simulink model "sampleModel10"  (R2021a)
settings: Solver=VariableStepAuto  StartTime=0.0  StopTime=10.0  RelTol=1e-3
undefined symbols (not defined in the file): Newton, Raphson
libraries: simulink x16, simulink_need_slupdate x4
settings Model: Creator=user  LastModifiedBy=user

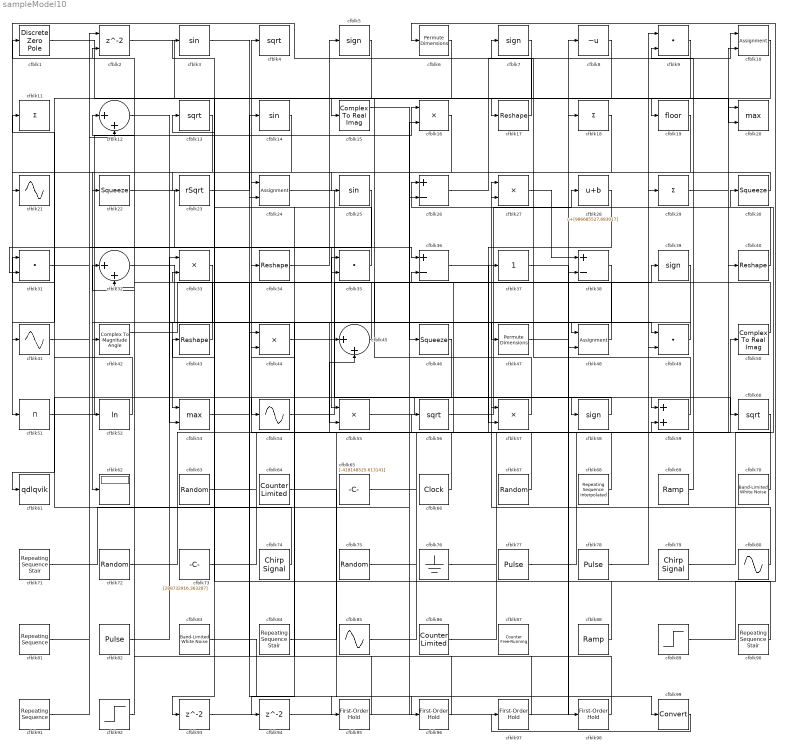
== system sampleModel10 ==
  cfblk1 : DiscreteZeroPole  Poles=[0 0.5]  Gain=1
  cfblk10 : Assignment  DiagnosticForDimensions=Warning  IndexOptions=Index vector (dialog)  Indices=1  OutputSizes=1
  cfblk11 : Sum  Inputs=+
  cfblk12 : Sum  Inputs=|++
  cfblk{4,13,56,60} (4 alike) : Sqrt  SaturateOnIntegerOverflow=on
  cfblk14 : Trigonometry
  cfblk15 : ComplexToRealImag
  cfblk{16,27,33,44,55} (5 alike) : Product
  cfblk{17,34,40,43} (4 alike) : Reshape
  cfblk18 : Sum  Inputs=+
  cfblk19 : Rounding
  cfblk2 : Delay  ShowEnablePort=on  SampleTime=1
      settings: InputPortMap=u0,e6
  cfblk20 : MinMax  Function=max  Inputs=2
  cfblk21 : Sin  TimeSource=Use external signal  SampleTime=0
  cfblk22 : Squeeze
  cfblk23 : Sqrt  Operator=rSqrt  AlgorithmType=Newton-Raphson  SaturateOnIntegerOverflow=on
  cfblk24 : Assignment  DiagnosticForDimensions=Warning  IndexOptions=Index vector (dialog)  Indices=1  OutputSizes=1
  cfblk25 : Trigonometry
  cfblk26 : Sum  Inputs=+-
  cfblk28 : Bias  Bias=[986685527.683017]
  cfblk29 : Sum  Inputs=+
  cfblk3 : Trigonometry
  cfblk30 : Squeeze
  cfblk{9,31,35,49} (4 alike) : DotProduct  InputSameDT=on  OutDataTypeStr=Inherit: Inherit via internal rule
  cfblk32 : Sum  Inputs=|++
  cfblk36 : Sum  Inputs=+-
  cfblk37 : simulink/Math Operations/Slider Gain  gain=1  low=0  high=2
  cfblk38 : Sum  Inputs=+-
  cfblk{5,7,39,58} (4 alike) : Signum
  cfblk41 : Sin  TimeSource=Use external signal  SampleTime=0
  cfblk42 : ComplexToMagnitudeAngle
  cfblk45 : Sum  Inputs=|++
  cfblk46 : Squeeze
  cfblk47 : PermuteDimensions
  cfblk48 : Assignment  DiagnosticForDimensions=Warning  IndexOptions=Index vector (dialog)  Indices=1  OutputSizes=1
  cfblk50 : ComplexToRealImag
  cfblk51 : Product  Inputs=*
  cfblk52 : Math  Operator=log  SaturateOnIntegerOverflow=on
  cfblk53 : MinMax  Function=max  Inputs=2
  cfblk54 : Sin  TimeSource=Use external signal  SampleTime=0
  cfblk57 : Product  Inputs=**
  cfblk59 : Sum
  cfblk6 : PermuteDimensions
  cfblk61 : ToWorkspace  VariableName=qdlqvik  SaveFormat=Timeseries  SampleTime=-1
  cfblk62 : Display
  cfblk63 : RandomNumber  Mean=[76846.263209]  Variance=[70057.951006]  Seed=[241872295.000000]  SampleTime=0.1
  cfblk64 : simulink/Sources/Counter Limited  uplimit=[760.000000]  tsamp=-1
  cfblk65 : Constant  Value=[-418148525.613141]  SampleTime=1
  cfblk66 : DigitalClock
  cfblk67 : UniformRandomNumber  Minimum=[-9938921969.734011]  Maximum=[3747111411.455578]  Seed=[43693278.000000]  SampleTime=0.1
  cfblk68 : simulink/Sources/Repeating Sequence Interpolated  OutValues=[-391403062.316644, -418279338.781921, -514967382.229999, 873367220.044669, 720380481.654073]  TimeValues=[0 0.1 0.5 0.6 1].'  LookUpMeth=Use Input Nearest  tsamp=0.01  OutMin=[]  OutMax=[]  OutDataTypeStr=double  OutputDataTypeScalingMode=double  OutDataType=fixdt(0,8)  OutScaling=2^-10
  cfblk69 : simulink/Sources/Ramp  slope=[-411.617913]  start=[28.684809]  InitialOutput=[-20761.220907]
  cfblk70 : simulink/Sources/Band-Limited White Noise  Cov=[2698116327.468347]  Ts=0.1  seed=[9897401420.000000]
  cfblk71 : simulink/Sources/Repeating Sequence Stair  OutValues=[-632648607.467752, 723313449.848045]  tsamp=-1  OutMin=[]  OutMax=[]  OutDataTypeStr=double  OutputDataTypeScalingMode=double  OutDataType=fixdt(0,8)  ConRadixGroup=Best Precision: Vector-wise  OutScaling=2^-12
  cfblk72 : RandomNumber  Mean=[-93473.485579]  Variance=[33195.801959]  Seed=[748746996.000000]  SampleTime=0.1
  cfblk73 : Constant  Value=[288732916.363287]  SampleTime=1
  cfblk74 : simulink/Sources/Chirp Signal  f1=[904410201.444868]  T=[86540470.784498]  f2=[-497173047.688361]
  cfblk75 : UniformRandomNumber  Minimum=[-4214276901.463890]  Maximum=[9154765990.333725]  Seed=[89559652.000000]  SampleTime=0.1
  cfblk76 : Ground
  cfblk77 : DiscretePulseGenerator  PulseType=Time based  Amplitude=[-34986765.239922]  Period=[44273998.333634]  PulseWidth=5  PhaseDelay=[3.000000]
  cfblk78 : DiscretePulseGenerator  PulseType=Time based  Amplitude=[-889372456.036665]  Period=[75379177.587079]  PulseWidth=5  PhaseDelay=[2.000000]
  cfblk79 : simulink/Sources/Chirp Signal  f1=[-288155761.833233]  T=[-208258071.970597]  f2=[771042454.979270]
  cfblk8 : UnaryMinus
  cfblk80 : Sin  Amplitude=[-957520902.756102]  Bias=[688161438.415493]  SampleTime=0
  cfblk81 : simulink/Sources/Repeating Sequence  rep_seq_t=[0 2]  rep_seq_y=[-423858712.355531, -499314234.927057]
  cfblk82 : DiscretePulseGenerator  PulseType=Time based  Amplitude=[-23240729.950069]  Period=[72903611.805465]  PulseWidth=5  PhaseDelay=[2.000000]
  cfblk83 : simulink/Sources/Band-Limited White Noise  Cov=[2162762055.148819]  Ts=0.1  seed=[9763345147.000000]
  cfblk84 : simulink/Sources/Repeating Sequence Stair  OutValues=[186471584.873103, -391192843.813065]  tsamp=-1  OutMin=[]  OutMax=[]  OutDataTypeStr=double  OutputDataTypeScalingMode=double  OutDataType=fixdt(0,8)  ConRadixGroup=Best Precision: Vector-wise  OutScaling=2^-12
  cfblk85 : Sin  Amplitude=[935405766.390659]  Bias=[791939661.303302]  SampleTime=0
  cfblk86 : simulink/Sources/Counter Limited  uplimit=[190.000000]  tsamp=-1
  cfblk87 : simulink/Sources/Counter Free-Running  NumBits=[1.000000]  tsamp=-1
  cfblk88 : simulink/Sources/Ramp  slope=[4235.275266]  start=[43.518613]  InitialOutput=[-763384.180324]
  cfblk89 : Step  Time=[2.000000]  Before=[196389050.859555]  After=[208627011.262656]  SampleTime=0
  cfblk90 : simulink/Sources/Repeating Sequence Stair  OutValues=[32864820.897776, -984985191.813432]  tsamp=-1  OutMin=[]  OutMax=[]  OutDataTypeStr=double  OutputDataTypeScalingMode=double  OutDataType=fixdt(0,8)  ConRadixGroup=Best Precision: Vector-wise  OutScaling=2^-12
  cfblk91 : simulink/Sources/Repeating Sequence  rep_seq_t=[0 2]  rep_seq_y=[377866727.176235, 892040750.789516]
  cfblk92 : Step  Time=[43.000000]  Before=[-773447094.952036]  After=[-290861317.614960]  SampleTime=0
  cfblk93 : Delay  SampleTime=1
  cfblk94 : Delay  SampleTime=1
  cfblk{95..98} (4 alike) : simulink_need_slupdate/First-Order Hold  DisableCoverage=on  Ts=1
      settings: SourceProductBaseCode=SL
  cfblk99 : DataTypeConversion
  wires:
  cfblk51/1 -> cfblk16/1
  cfblk27/1 -> cfblk38/1
  cfblk75/1 -> cfblk50/1
  cfblk32/1 -> cfblk48/1
  cfblk67/1 -> cfblk4/1
  cfblk14/1 -> cfblk62/1
  cfblk85/1 -> cfblk8/1
  cfblk79/1 -> cfblk30/1
  cfblk17/1 -> cfblk51/1
  cfblk72/1 -> cfblk38/2
  cfblk46/1 -> cfblk61/1
  cfblk18/1 -> cfblk21/1
  cfblk54/1 -> cfblk39/1
  cfblk15/1 -> cfblk46/1
  cfblk13/1 -> cfblk22/1
  cfblk33/1 -> cfblk53/1
  cfblk1/1 -> cfblk17/1
  cfblk47/1 -> cfblk49/1
  cfblk82/1 -> cfblk33/1
  cfblk52/1 -> cfblk11/1
  cfblk55/1 -> cfblk59/1
  cfblk91/1 -> cfblk52/1
  cfblk22/1 -> cfblk55/1
  cfblk41/1 -> cfblk2/1
  cfblk43/1 -> cfblk1/1
  cfblk24/1 -> cfblk58/1
  cfblk40/1 -> cfblk26/1
  cfblk78/1 -> cfblk49/2
  cfblk36/1 -> cfblk28/1
  cfblk70/1 -> cfblk56/1
  cfblk88/1 -> cfblk43/1
  cfblk74/1 -> cfblk31/1
  cfblk80/1 -> cfblk27/1
  cfblk66/1 -> cfblk24/1
  cfblk44/1 -> cfblk60/1
  cfblk16/1 -> cfblk25/1
  cfblk9/1 -> cfblk19/1
  cfblk30/1 -> cfblk23/1
  cfblk77/1 -> cfblk20/1
  cfblk48/1 -> cfblk33/2
  cfblk10/1 -> cfblk45/1
  cfblk31/1 -> cfblk36/1
  cfblk56/1 -> cfblk18/1
  cfblk19/1 -> cfblk53/2
  cfblk86/1 -> cfblk40/1
  cfblk26/1 -> cfblk10/1
  cfblk84/1 -> cfblk29/1
  cfblk25/1 -> cfblk31/2
  cfblk57/1 -> cfblk34/1
  cfblk2/1 -> cfblk20/2
  cfblk49/1 -> cfblk42/1
  cfblk7/1 -> cfblk15/1
  cfblk23/1 -> cfblk14/1
  cfblk76/1 -> cfblk9/1
  cfblk6/1 -> cfblk24/2
  cfblk71/1 -> cfblk26/2
  cfblk89/1 -> cfblk6/1
  cfblk35/1 -> cfblk13/1
  cfblk69/1 -> cfblk9/2
  cfblk90/1 -> cfblk3/1
  cfblk29/1 -> cfblk10/2
  cfblk12/1 -> cfblk47/1
  cfblk65/1 -> cfblk37/1
  cfblk63/1 -> cfblk57/1
  cfblk45/1 -> cfblk12/1
  cfblk81/1 -> cfblk12/2
  cfblk73/1 -> cfblk45/2
  cfblk39/1 -> cfblk55/2
  cfblk59/1 -> cfblk27/2
  cfblk60/1 -> cfblk59/2
  cfblk58/1 -> cfblk54/1
  cfblk68/1 -> cfblk36/2
  cfblk92/1 -> cfblk2/2
  cfblk34/1 -> cfblk5/1
  cfblk8/1 -> cfblk41/1
  cfblk28/1 -> cfblk57/2
  cfblk42/1 -> cfblk35/1
  cfblk53/1 -> cfblk35/2
  cfblk50/1 -> cfblk7/1
  cfblk5/1 -> cfblk93/1
  cfblk93/1 -> cfblk16/2
  cfblk38/1 -> cfblk94/1
  cfblk94/1 -> cfblk48/2
  cfblk3/1 -> cfblk95/1
  cfblk95/1 -> cfblk32/1
  cfblk83/1 -> cfblk96/1
  cfblk96/1 -> cfblk32/2
  cfblk97/1 -> cfblk44/1
  cfblk37/1 -> cfblk98/1
  cfblk98/1 -> cfblk44/2
  cfblk64/1 -> cfblk99/1
  cfblk99/1 -> cfblk97/1
